simulink model "FOC_Ctrl_CodeModel"  (R2020b)
settings: Solver=FixedStepDiscrete  StartTime=0.0  StopTime=10.0  FixedStep=Ts  RelTol=1e-3
values from neighbouring files (symbols this model uses):
  EstOutMax_Speed = 2.0    (= 2)    [FOC_Config.m]
  fluxF = Lam_realvalue/fluxB    [FOC_Config.m]
  Ld = Ld_realvalue/Lb    [FOC_Config.m]
  Lq = Lq_realvalue/Lb    [FOC_Config.m]
  Omega0 = 0.4    [PLLObserver.sldd]
  PLL_KI = PLL_Bandwidth*PLL_Bandwidth    (= 0.16)    [FOC_Config.m]
  PLL_KP = 2*PLL_Bandwidth    (= 0.8)    [FOC_Config.m]
  PLL_OUTMax_W = 1.2    [FOC_Config.m]
  Rs = Rs_realvalue/Rb    [FOC_Config.m]
  SVCM_GAIN = 0.8    [FOC_Config.m]
  tb = 1/Wb    (= 0.000636619772368)    [FOC_Config.m]
undefined symbols (not defined in the file or in its folder): DiscIntNeverNeededParam, EstOutMax_Theta
settings Model: DataDictionary=PLLObserver.sldd  Creator=k  LastModifiedBy=wangdi
settings OptimizationCC: DefaultParameterBehavior=Inlined  GainParamInheritBuiltInType=on  UseFloatMulNetSlope=on  DefaultUnderspecifiedDataType=single  UseSpecifiedMinMax=on  InlineInvariantSignals=on  BitwiseOrLogicalOp=Bitwise operator  PassReuseOutputArgsAs=Individual arguments  ZeroExternalMemoryAtStartup=off  ZeroInternalMemoryAtStartup=off  NoFixptDivByZeroProtection=on  EfficientFloat2IntCast=on  OptimizeBlockOrder=speed  DifferentSizesBufferReuse=on  EfficientTunableParamExpr=on
settings DebuggingCC: ParameterTunabilityLossMsg=error
settings HardwareCC: ProdLongLongMode=on
settings SFSimCC: MATLABDynamicMemAlloc=off
settings RTWCC: Description=Embedded Coder  SystemTargetFile=ert.tlc  GenCodeOnly=on  TemplateMakefile=ert_default_tmf  GenerateReport=on  BuildConfiguration=Faster Runs  LaunchReport=on  GenerateCodeMetricsReport=on
settings CodeAppCC: ForceParamTrailComments=on  IgnoreCustomStorageClasses=off  OperatorAnnotations=on  SimulinkDataObjDesc=on  SFDataObjDesc=on  InsertBlockDesc=on
settings ERTTargetCC: TargetLangStandard=C99 (ISO)  UtilityFuncGeneration=Shared location  GenerateSampleERTMain=on  IncludeMdlTerminateFcn=off  CombineSignalStateStructs=on  SuppressErrorStatus=on  SupportNonFinite=off  InlinedParameterPlacement=NonHierarchical  ERTCustomFileTemplate=example_file_process.tlc

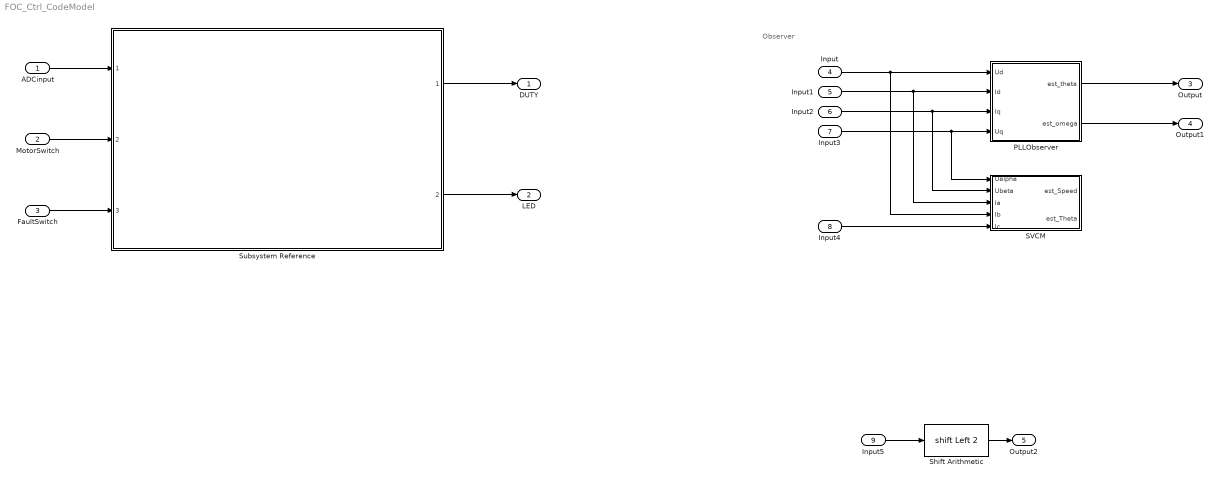
== system FOC_Ctrl_CodeModel ==
  note: Observer
  ADCinput : Inport  OutDataTypeStr=uint16  PortDimensions=5
  MotorSwitch : Inport  Port=2  OutDataTypeStr=boolean  PortDimensions=1
  FaultSwitch : Inport  Port=3  OutDataTypeStr=boolean  PortDimensions=1
  Input : Inport  Port=4
  Input1 : Inport  Port=5
  Input2 : Inport  Port=6  OutDataTypeStr=single
  Input3 : Inport  Port=7  OutDataTypeStr=single
  Input4 : Inport  Port=8  OutDataTypeStr=single
  Input5 : Inport  Port=9  OutDataTypeStr=int16
  PLLObserver : Subsystem  TreatAsAtomicUnit=on
      settings: RTWFcnNameOpts=Use subsystem name  RTWFileNameOpts=Use subsystem name
  SVCM : Subsystem  TreatAsAtomicUnit=on
      settings: RTWFcnNameOpts=Use subsystem name  RTWFileNameOpts=Use subsystem name
  Shift Arithmetic : ArithShift  BitShiftNumber=2  BitShiftDirection=Left
  Subsystem Reference : Subsystem  ReferencedSubsystem=FOC_Sub_StateMch
  DUTY : Outport  PortDimensions=3
  LED : Outport  Port=2  PortDimensions=3
  Output : Outport  Port=3
  Output1 : Outport  Port=4
  Output2 : Outport  Port=5  OutDataTypeStr=int16
  wires:
  FaultSwitch/1 -> Subsystem Reference/3
  MotorSwitch/1 -> Subsystem Reference/2
  ADCinput/1 -> Subsystem Reference/1
  Subsystem Reference/1 -> DUTY/1
  Subsystem Reference/2 -> LED/1
  Input3/1 -> SVCM/1(Ualpha), PLLObserver/4(Uq)
  Input2/1 -> SVCM/2(Ubeta), PLLObserver/3(Iq)
  Input/1 -> SVCM/4(Ib), PLLObserver/1(Ud)
  Input1/1 -> SVCM/3(Ia), PLLObserver/2(Id)
  PLLObserver/2(est_omega) -> Output1/1
  PLLObserver/1(est_theta) -> Output/1
  Input4/1 -> SVCM/5(Ic)
  Input5/1 -> Shift Arithmetic/1
  Shift Arithmetic/1 -> Output2/1

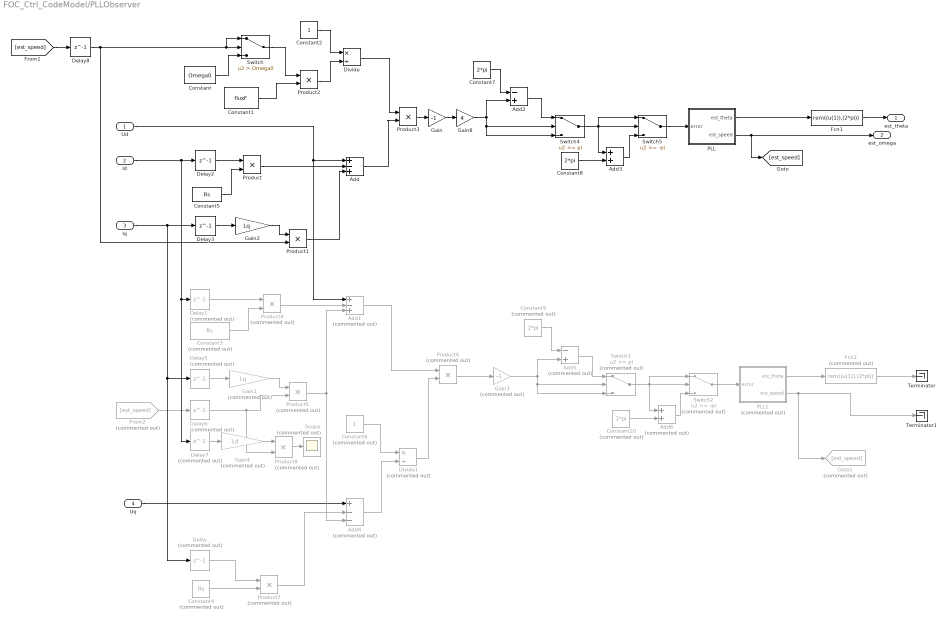
== system FOC_Ctrl_CodeModel/PLLObserver ==
  Ud : Inport
  Id : Inport  Port=2
  Iq : Inport  Port=3
  Uq : Inport  Port=4
  Add : Sum  Inputs=+-+
  Add1 : Sum  Commented=on  Inputs=+-+
  Add2 : Sum  Inputs=-+
  Add3 : Sum
  Add4 : Sum  Commented=on  Inputs=+--
  Add5 : Sum  Commented=on  Inputs=-+
  Add6 : Sum  Commented=on
  Constant : Constant  Value=Omega0  OutDataTypeStr=single
  Constant1 : Constant  Value=fluxF  OutDataTypeStr=single
  Constant10 : Constant  Commented=on  Value=2*pi
  Constant2 : Constant  OutDataTypeStr=single
  Constant3 : Constant  Commented=on  Value=Rs  OutDataTypeStr=single
  Constant4 : Constant  Commented=on  Value=Rs  OutDataTypeStr=single
  Constant5 : Constant  Value=Rs  OutDataTypeStr=single
  Constant6 : Constant  Commented=on  OutDataTypeStr=single
  Constant7 : Constant  Value=2*pi  OutDataTypeStr=single
  Constant8 : Constant  Value=2*pi  OutDataTypeStr=single
  Constant9 : Constant  Commented=on  Value=2*pi  OutDataTypeStr=single
  Delay{,1,5..7} (5 alike) : Delay  Commented=on  DelayLength=1
  Delay2 : Delay  DelayLength=1
  Delay3 : Delay  DelayLength=1
  Delay8 : Delay  DelayLength=1
  Divide : Product  Inputs=*/
  Divide1 : Product  Commented=on  Inputs=*/
  Fcn1 : Fcn  Expr=rem((u(1)),(2*pi))
  Fcn2 : Fcn  Commented=on  Expr=rem((u(1)),(2*pi))
  From2 : From  Commented=on  GotoTag=est_speed
  Gain : Gain  Gain=-1
  Gain1 : Gain  Commented=on  Gain=Lq
  Gain2 : Gain  Gain=Lq
  Gain3 : Gain  Commented=on  Gain=-1
  Gain4 : Gain  Commented=on  Gain=Ld
  Gain8 : Gain  Gain=4
  Goto1 : Goto  Commented=on  GotoTag=est_speed
  PLL : Subsystem
  PLL1 : Subsystem  Commented=on
  Product{,1..3} (4 alike) : Product
  Product{4..8} (5 alike) : Product  Commented=on
  Scope : Scope  Commented=on
  Switch : Switch  Criteria=u2 > Threshold  Threshold=Omega0
  Switch1 : Switch  Commented=on  Threshold=pi
  Switch2 : Switch  Commented=on  Threshold=-pi
  Switch4 : Switch  Threshold=pi
  Switch5 : Switch  Threshold=-pi
  Terminator : Terminator
  Terminator1 : Terminator
  est_theta : Outport
  est_omega : Outport  Port=2
  wires:
  [est_speed] -> Delay8/1
  PLL/1(est_theta) -> Fcn1/1
  Gain8/1 -> Add2/2, Switch4/2, Switch4/3
  Add/1 -> Product3/2
  Product1/1 -> Add/3
  Product/1 -> Add/2
  Product8/1 -> Scope/1
  Gain4/1 -> Product8/1
  From2/1 -> Delay6/1
  Delay7/1 -> Gain4/1
  Fcn1/1 -> est_theta/1
  PLL1/2(est_speed) -> Goto1/1, Terminator1/1
  Fcn2/1 -> Terminator/1
  PLL1/1(est_theta) -> Fcn2/1
  Add6/1 -> Switch2/3
  Gain3/1 -> Add5/2, Switch1/2, Switch1/3
  Add5/1 -> Switch1/1
  Switch2/1 -> PLL1/1(error)
  Constant10/1 -> Add6/2
  Constant9/1 -> Add5/1
  Switch1/1 -> Switch2/2, Add6/1, Switch2/1
  Product6/1 -> Gain3/1
  Divide1/1 -> Product6/2
  Add4/1 -> Divide1/2
  Constant6/1 -> Divide1/1
  Product7/1 -> Add4/2
  Constant4/1 -> Product7/2
  Delay/1 -> Product7/1
  Uq/1 -> Add4/1
  Add1/1 -> Product6/1
  Product5/1 -> Add1/3, Add4/3
  Iq/1 -> Delay3/1, Delay5/1, Delay/1
  Delay5/1 -> Gain1/1
  Gain1/1 -> Product5/1
  Delay6/1 -> Product5/2, Product8/2
  Ud/1 -> Add/1, Add1/1
  Delay1/1 -> Product4/1
  Product4/1 -> Add1/2
  Constant3/1 -> Product4/2
  Gain/1 -> Gain8/1
  Product3/1 -> Gain/1
  Switch5/1 -> PLL/1(error)
  Add2/1 -> Switch4/1
  Constant7/1 -> Add2/1
  Constant8/1 -> Add3/2
  Add3/1 -> Switch5/3
  PLL/2(est_speed) -> [est_speed], est_omega/1
  Switch4/1 -> Switch5/2, Add3/1, Switch5/1
  Divide/1 -> Product3/1
  Product2/1 -> Divide/2
  Constant2/1 -> Divide/1
  Constant1/1 -> Product2/2
  Switch/1 -> Product2/1
  Constant/1 -> Switch/3
  Id/1 -> Delay2/1, Delay1/1, Delay7/1
  Delay2/1 -> Product/1
  Delay3/1 -> Gain2/1
  Gain2/1 -> Product1/1
  Delay8/1 -> Switch/2, Switch/1, Product1/2
  Constant5/1 -> Product/2

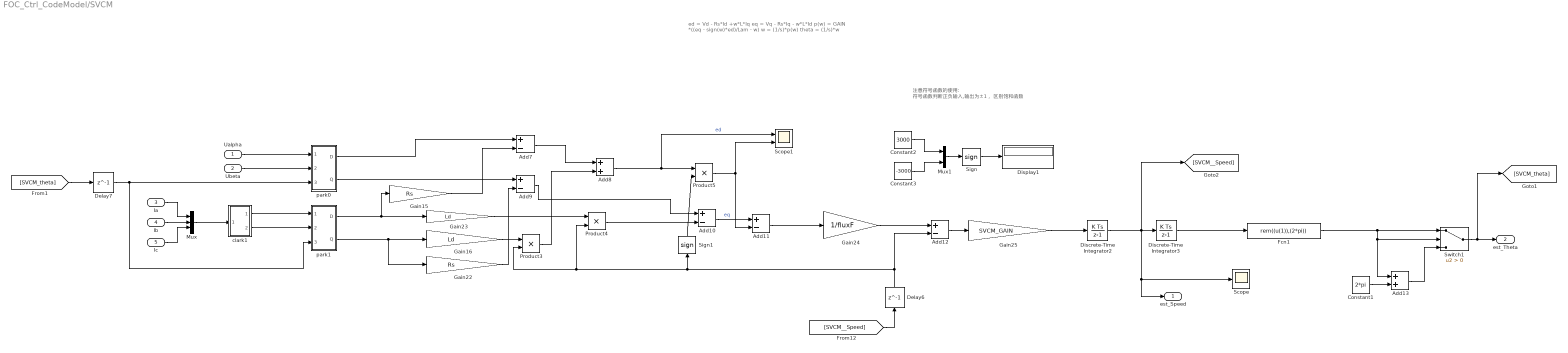
== system FOC_Ctrl_CodeModel/SVCM ==
  note: 注意符号函数的使用:
      | 符号函数判断正负输入,输出为±1，
      | 区别饱和函数
  note: ed = Vd - Rs*Id +w*L*Iq
      | eq = Vq - Rs*Iq - w*L*Id
      | p(w) = GAIN *((eq - sign(w)*ed)/Lam - w)
      | w = (1/s)*p(w)
      | theta = (1/s)*w
  Ualpha : Inport  OutDataTypeStr=single
  Ubeta : Inport  Port=2  OutDataTypeStr=single
  Ia : Inport  Port=3
  Ib : Inport  Port=4
  Ic : Inport  Port=5
  Add{7,9..12} (5 alike) : Sum  Inputs=+-
  Add13 : Sum
  Add8 : Sum
  Constant1 : Constant  Value=2*pi
  Constant2 : Constant  Value=3000
  Constant3 : Constant  Value=-3000
  Delay6 : Delay  DelayLength=1
  Delay7 : Delay  DelayLength=1
  Discrete-Time Integrator2 : DiscreteIntegrator  gainval=1.0/tb  SampleTime=-1  LimitOutput=on  UpperSaturationLimit=EstOutMax_Speed  LowerSaturationLimit=-EstOutMax_Speed  ICPrevOutput=DiscIntNeverNeededParam  ICPrevScaledInput=DiscIntNeverNeededParam
  Discrete-Time Integrator3 : DiscreteIntegrator  gainval=1.0/tb  SampleTime=-1  UpperSaturationLimit=EstOutMax_Theta  LowerSaturationLimit=-EstOutMax_Theta  ICPrevOutput=DiscIntNeverNeededParam  ICPrevScaledInput=DiscIntNeverNeededParam
  Display1 : Display
      settings: Decimation=2
  Fcn1 : Fcn  Expr=rem((u(1)),(2*pi))
  Gain15 : Gain  Gain=Rs
  Gain16 : Gain  Gain=Ld
  Gain22 : Gain  Gain=Rs
  Gain23 : Gain  Gain=Ld
  Gain24 : Gain  Gain=1/fluxF
  Gain25 : Gain  Gain=SVCM_GAIN
  Mux : Mux  Inputs=3
  Mux1 : Mux  Inputs=2
  Product3 : Product
  Product4 : Product
  Product5 : Product
  Scope : Scope
  Scope1 : Scope  NumInputPorts=2
  Sign : Signum
  Sign1 : Signum
  Switch1 : Switch  Criteria=u2 > Threshold
  clark1 : Subsystem
  park0 : Subsystem
  park1 : Subsystem
  est_Speed : Outport  OutDataTypeStr=single
  est_Theta : Outport  Port=2  OutDataTypeStr=single
  wires:
  Gain15/1 -> Add7/2
  Gain22/1 -> Add9/2
  Switch1/1 -> est_Theta/1, [SVCM_theta]
  Add13/1 -> Switch1/3
  Ualpha/1 -> park0/1(alpha)
  Ubeta/1 -> park0/2(beta)
  Delay7/1 -> park0/3(theta), park1/3(theta)
  [SVCM_theta] -> Delay7/1
  clark1/2(Ibeta) -> park1/2(beta)
  [SVCM__Speed] -> Delay6/1
  clark1/1(Ialpha) -> park1/1(alpha)
  Add12/1 -> Gain25/1
  Add7/1 -> Add8/1
  Add10/1 -> Add11/1  "eq"
  Add8/1 -> Scope1/1, Product5/1  "ed"
  Constant1/1 -> Add13/2
  Gain24/1 -> Add12/1
  Gain16/1 -> Product3/1
  Add9/1 -> Add10/1
  Gain23/1 -> Product4/1
  Delay6/1 -> Product4/2, Product3/2, Sign1/1, Add12/2
  Mux/1 -> clark1/1(Iabc)
  Discrete-Time Integrator3/1 -> Fcn1/1
  Fcn1/1 -> Switch1/1, Add13/1, Switch1/2
  Discrete-Time Integrator2/1 -> Scope/1, est_Speed/1, [SVCM__Speed], Discrete-Time Integrator3/1
  Product3/1 -> Add8/2
  Product4/1 -> Add10/2
  Product5/1 -> Add11/2, Scope1/2
  Sign1/1 -> Product5/2
  Add11/1 -> Gain24/1
  Gain25/1 -> Discrete-Time Integrator2/1
  Sign/1 -> Display1/1
  Constant2/1 -> Mux1/1
  Constant3/1 -> Mux1/2
  Mux1/1 -> Sign/1
  park0/1(D) -> Add7/1
  park0/2(Q) -> Add9/1
  park1/1(D) -> Gain23/1, Gain15/1
  park1/2(Q) -> Gain22/1, Gain16/1
  Ia/1 -> Mux/1
  Ib/1 -> Mux/2
  Ic/1 -> Mux/3

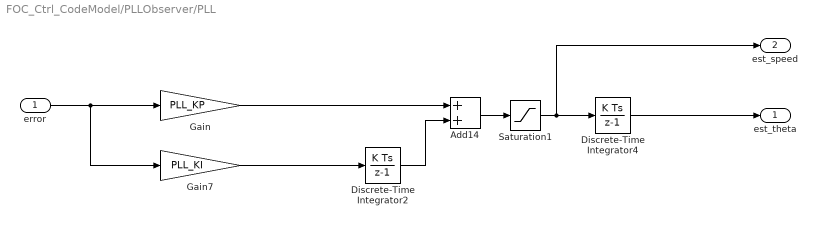
== system FOC_Ctrl_CodeModel/PLLObserver/PLL ==
  error : Inport
  Add14 : Sum
  Discrete-Time Integrator2 : DiscreteIntegrator  gainval=1/tb  SampleTime=-1  LimitOutput=on  UpperSaturationLimit=PLL_OUTMax_W  LowerSaturationLimit=-PLL_OUTMax_W  ICPrevOutput=DiscIntNeverNeededParam  ICPrevScaledInput=DiscIntNeverNeededParam
  Discrete-Time Integrator4 : DiscreteIntegrator  gainval=1.0/tb  SampleTime=-1  UpperSaturationLimit=PLL_OUTMax_W  LowerSaturationLimit=-PLL_OUTMax_W  ICPrevOutput=DiscIntNeverNeededParam  ICPrevScaledInput=DiscIntNeverNeededParam
  Gain : Gain  Gain=PLL_KP
  Gain7 : Gain  Gain=PLL_KI
  Saturation1 : Saturate  UpperLimit=PLL_OUTMax_W  LowerLimit=-PLL_OUTMax_W
  est_theta : Outport
  est_speed : Outport  Port=2
  wires:
  Discrete-Time Integrator4/1 -> est_theta/1
  Gain7/1 -> Discrete-Time Integrator2/1
  Gain/1 -> Add14/1
  Discrete-Time Integrator2/1 -> Add14/2
  error/1 -> Gain/1, Gain7/1
  Saturation1/1 -> Discrete-Time Integrator4/1, est_speed/1
  Add14/1 -> Saturation1/1

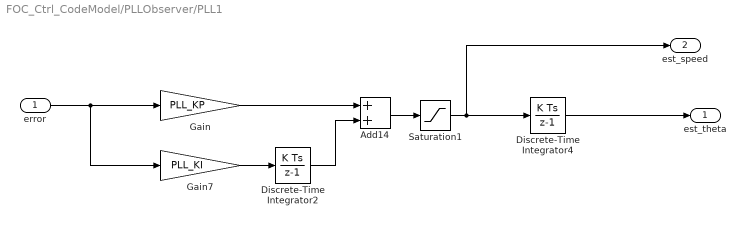
== system FOC_Ctrl_CodeModel/PLLObserver/PLL1 ==
  error : Inport
  Add14 : Sum
  Discrete-Time Integrator2 : DiscreteIntegrator  gainval=1.0/tb  SampleTime=-1  LimitOutput=on  UpperSaturationLimit=PLL_OUTMax_W  LowerSaturationLimit=-PLL_OUTMax_W  ICPrevOutput=DiscIntNeverNeededParam  ICPrevScaledInput=DiscIntNeverNeededParam
  Discrete-Time Integrator4 : DiscreteIntegrator  gainval=1.0/tb  SampleTime=-1  UpperSaturationLimit=PLL_OUTMax_W  LowerSaturationLimit=-PLL_OUTMax_W  ICPrevOutput=DiscIntNeverNeededParam  ICPrevScaledInput=DiscIntNeverNeededParam
  Gain : Gain  Gain=PLL_KP
  Gain7 : Gain  Gain=PLL_KI
  Saturation1 : Saturate  UpperLimit=PLL_OUTMax_W  LowerLimit=-PLL_OUTMax_W
  est_theta : Outport
  est_speed : Outport  Port=2
  wires:
  Gain/1 -> Add14/1
  Discrete-Time Integrator2/1 -> Add14/2
  error/1 -> Gain/1, Gain7/1
  Saturation1/1 -> Discrete-Time Integrator4/1, est_speed/1
  Add14/1 -> Saturation1/1
  Discrete-Time Integrator4/1 -> est_theta/1
  Gain7/1 -> Discrete-Time Integrator2/1

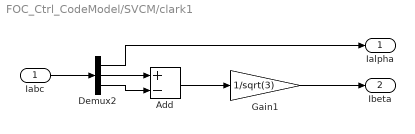
== system FOC_Ctrl_CodeModel/SVCM/clark1 ==
  Iabc : Inport
  Add : Sum  Inputs=+-
  Demux2 : Demux  Outputs=3
  Gain1 : Gain  Gain=1/sqrt(3)
  Ialpha : Outport
  Ibeta : Outport  Port=2
  wires:
  Demux2/3 -> Add/2
  Demux2/1 -> Ialpha/1
  Demux2/2 -> Add/1
  Iabc/1 -> Demux2/1
  Add/1 -> Gain1/1
  Gain1/1 -> Ibeta/1

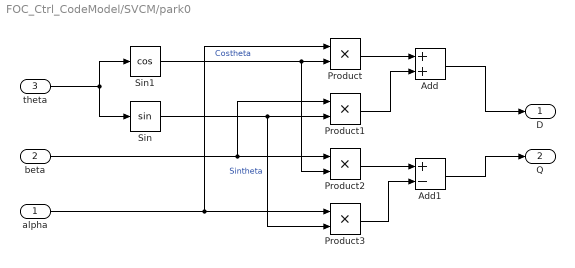
== system FOC_Ctrl_CodeModel/SVCM/park0 ==
  alpha : Inport
  beta : Inport  Port=2
  theta : Inport  Port=3
  Add : Sum
  Add1 : Sum  Inputs=+-
  Product{,1..3} (4 alike) : Product
  Sin : Trigonometry
  Sin1 : Trigonometry  Operator=cos
  D : Outport
  Q : Outport  Port=2
  wires:
  theta/1 -> Sin1/1, Sin/1
  Product2/1 -> Add1/1
  Sin/1 -> Product1/2, Product3/2  "Sintheta"
  Add/1 -> D/1
  Product3/1 -> Add1/2
  Sin1/1 -> Product2/2, Product/2  "Costheta"
  beta/1 -> Product1/1, Product2/1
  Product1/1 -> Add/2
  Product/1 -> Add/1
  alpha/1 -> Product/1, Product3/1
  Add1/1 -> Q/1

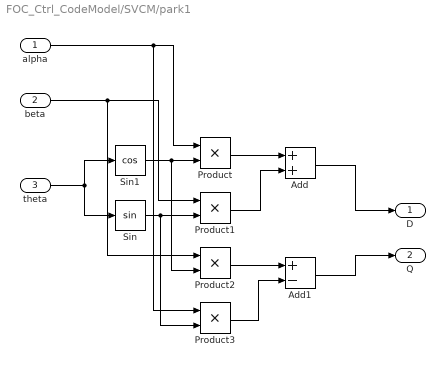
== system FOC_Ctrl_CodeModel/SVCM/park1 ==
  alpha : Inport
  beta : Inport  Port=2
  theta : Inport  Port=3
  Add : Sum
  Add1 : Sum  Inputs=+-
  Product{,1..3} (4 alike) : Product
  Sin : Trigonometry
  Sin1 : Trigonometry  Operator=cos
  D : Outport
  Q : Outport  Port=2
  wires:
  Add1/1 -> Q/1
  alpha/1 -> Product/1, Product3/1
  Product/1 -> Add/1
  Product1/1 -> Add/2
  beta/1 -> Product2/1, Product1/1
  Sin1/1 -> Product/2, Product2/2
  Product3/1 -> Add1/2
  Add/1 -> D/1
  Sin/1 -> Product1/2, Product3/2
  Product2/1 -> Add1/1
  theta/1 -> Sin/1, Sin1/1
